simulink model "zad12_test"  (R2014b)
settings: Solver=ode45  StartTime=0.0  StopTime=70  RelTol=1e-3
values from neighbouring files (symbols this model uses):
  a1 = -0.28    [set_params.m]
  a2 = -0.9    [set_params.m]
  a3 = 0.35    [set_params.m]
  a4 = 0.3    [set_params.m]
  K = 4.5    [set_params.m]
  T1 = 5    [set_params.m]
  T2 = 8    [set_params.m]
  u_lin = linspace(-1,1,101)    [zad11.m]    (also in zad12.m = 1; zad6.m = K*a1*u + K*(a2*(u_p^2) + a3*(u_p^3) + a4*(u_p^4)) + K*(u - u; zad9.m = pkt_lin(i))
settings Model: Creator=kuba  LastModifiedBy=kuba
settings DebuggingCC: SolverPrmCheckMsg=none

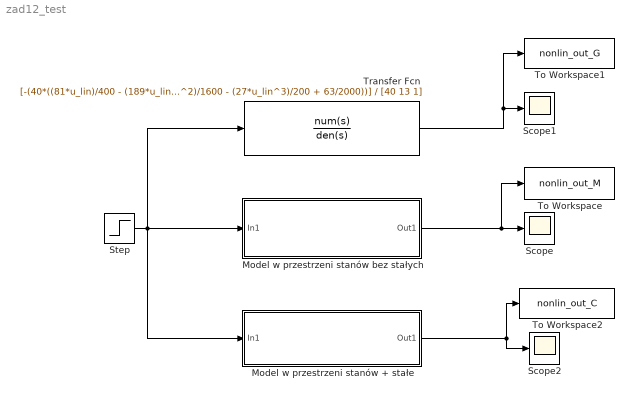
== system zad12_test ==
  Model w przestrzeni stanów + stałe : Subsystem
  "Model w przestrzeni stanów bez stałych " : Subsystem
  Scope : Scope
  Scope1 : Scope
  Scope2 : Scope
      settings: SaveName=ScopeData2
  Step : Step  SampleTime=0
  To Workspace : ToWorkspace  VariableName=nonlin_out_M  SaveFormat=Timeseries  SampleTime=-1
  To Workspace1 : ToWorkspace  VariableName=nonlin_out_G  SaveFormat=Timeseries  SampleTime=-1
  To Workspace2 : ToWorkspace  VariableName=nonlin_out_C  SaveFormat=Timeseries  SampleTime=-1
  Transfer Fcn : TransferFcn  Numerator=[-(40*((81*u_lin)/400 - (189*u_lin^2)/1600 - (27*u_lin^3)/200 + 63/2000))]  Denominator=[40 13 1]
  wires:
  Transfer Fcn/1 -> To Workspace1/1, Scope1/1
  "Model w przestrzeni stanów bez stałych "/1(Out1) -> To Workspace/1, Scope/1
  Step/1 -> Model w przestrzeni stanów + stałe/1(In1), "Model w przestrzeni stanów bez stałych "/1(In1), Transfer Fcn/1
  Model w przestrzeni stanów + stałe/1(Out1) -> Scope2/1, To Workspace2/1

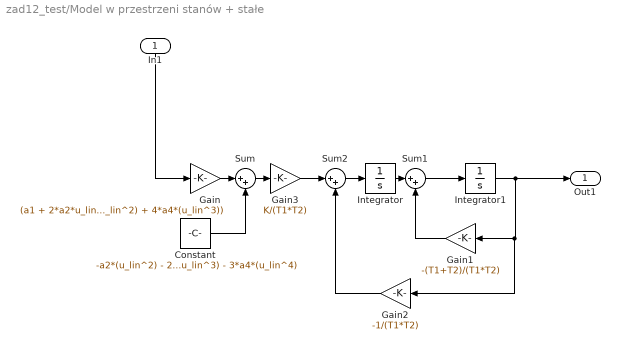
== system zad12_test/Model w przestrzeni stanów + stałe ==
  In1 : Inport
  Constant : Constant  Value=-a2*(u_lin^2) - 2*a3*(u_lin^3) - 3*a4*(u_lin^4)
  Gain : Gain  Gain=(a1 + 2*a2*u_lin + 3*a3*(u_lin^2) + 4*a4*(u_lin^3))
  Gain1 : Gain  Gain=-(T1+T2)/(T1*T2)
  Gain2 : Gain  Gain=-1/(T1*T2)
  Gain3 : Gain  Gain=K/(T1*T2)
  Integrator : Integrator
  Integrator1 : Integrator
  Sum : Sum  Inputs=|++
  Sum1 : Sum  Inputs=|++
  Sum2 : Sum  Inputs=|++
  Out1 : Outport
  wires:
  Gain/1 -> Sum/1
  Integrator/1 -> Sum1/1
  Sum1/1 -> Integrator1/1
  Sum2/1 -> Integrator/1
  Gain1/1 -> Sum1/2
  Constant/1 -> Sum/2
  Gain2/1 -> Sum2/2
  Gain3/1 -> Sum2/1
  Sum/1 -> Gain3/1
  Integrator1/1 -> Out1/1, Gain2/1, Gain1/1
  In1/1 -> Gain/1

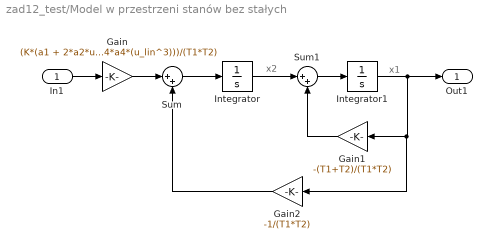
== system zad12_test/Model w przestrzeni stanów bez stałych  ==
  note: x2
  note: x1
  In1 : Inport
  Gain : Gain  Gain=(K*(a1 + 2*a2*u_lin + 3*a3*(u_lin^2) + 4*a4*(u_lin^3)))/(T1*T2)
  Gain1 : Gain  Gain=-(T1+T2)/(T1*T2)
  Gain2 : Gain  Gain=-1/(T1*T2)
  Integrator : Integrator
  Integrator1 : Integrator
  Sum : Sum  Inputs=|++
  Sum1 : Sum  Inputs=|++
  Out1 : Outport
  wires:
  Gain/1 -> Sum/1
  Sum/1 -> Integrator/1
  Integrator/1 -> Sum1/1
  Sum1/1 -> Integrator1/1
  Integrator1/1 -> Out1/1, Gain2/1, Gain1/1
  Gain1/1 -> Sum1/2
  Gain2/1 -> Sum/2
  In1/1 -> Gain/1
